simulink model "modelo_matematico"  (R2018b)
settings: Solver=ode4  StartTime=0.0  StopTime=t_f  FixedStep=fst  RelTol=1e-3  EnableMultiTasking=on
values from neighbouring files (symbols this model uses):
  a = plot(dado_t, dado_vd, '-', 'Color',[1.0,0.5,0.0], 'LineWidth', 4)    [Graficos.m]    (also in Trajetoria_Curva_180_graus_RAMPA.m = 0.15)
  b = plot(dado_t, dado_vr, '-', 'Color',[0.0,0.0,0.0], 'LineWidth', 1)    [Graficos.m]    (also in script_principal.m = 0.121)
  c_d = r_d/(2*b)    (= 0.120661157025)    [script_principal.m]
  c_e = r_e/(2*b)    (= 0.121074380165)    [script_principal.m]
  dur_c = dist_c/v    (= 3.5903916041)    [Trajetoria_Curva_180_graus_RAMPA.m]
  k0 = 10    [script_principal.m]
  KaD = 0.4713    [script_principal.m]
  KaD_v = var_KaD*0.4713    (= 0.4713)    [script_principal.m]
  KaE = 0.5046    [script_principal.m]
  KaE_v = var_KaE*0.5046    (= 0.5046)    [script_principal.m]
  L = 0.1    [script_principal.m]
  T = 3    [script_principal.m]
  t_f = t_i+dur_0+dur_1+dur_c+dur_2+dur_3    (= 17.9237249374)    [Trajetoria_Curva_180_graus_RAMPA.m]
  t_i = 0    [Trajetoria_Curva_180_graus_RAMPA.m]
  t_i_1 = t_i+dur_0    (= 2.33333333333)    [Trajetoria_Curva_180_graus_RAMPA.m]
  t_i_2 = t_i+dur_0+dur_1+dur_c    (= 10.7570582708)    [Trajetoria_Curva_180_graus_RAMPA.m]
  t_i_3 = t_i+dur_0+dur_1+dur_c+dur_2    (= 15.5903916041)    [Trajetoria_Curva_180_graus_RAMPA.m]
  t_i_c = t_i+dur_0+dur_1    (= 7.16666666667)    [Trajetoria_Curva_180_graus_RAMPA.m]
  v = 0.35    [Trajetoria_Curva_180_graus_RAMPA.m]
  VaD_max = 14    [script_principal.m]
  VaE_max = 14    [script_principal.m]
  x0 = [x0_1; x0_2; x0_3]    [script_principal.m]
undefined symbols (not defined in the file or in its folder): time_c, w, wx, wy
libraries: simulink x37, dspmtrx3 x2
settings Model: Creator=nenem  LastModifiedBy=nenem
settings OptimizationCC: LifeSpan=inf
settings DebuggingCC: SFUnexpectedBacktrackingDiag=warning  SFNoUnconditionalDefaultTransitionDiag=warning
settings SFSimCC: SimUseLocalCustomCode=off
settings RTWCC: RTWUseLocalCustomCode=off
settings CodeAppCC: StateflowObjectComments=on
settings GRTTargetCC: TargetLangStandard=C89/C90 (ANSI)  GeneratePreprocessorConditionals=Disable all
settings ConfigComp: CovMetricSettings=dw  CovHtmlReporting=on  CovSaveCumulativeToWorkspaceVar=on  CovSaveSingleToWorkspaceVar=on  CovExternalEMLEnable=off

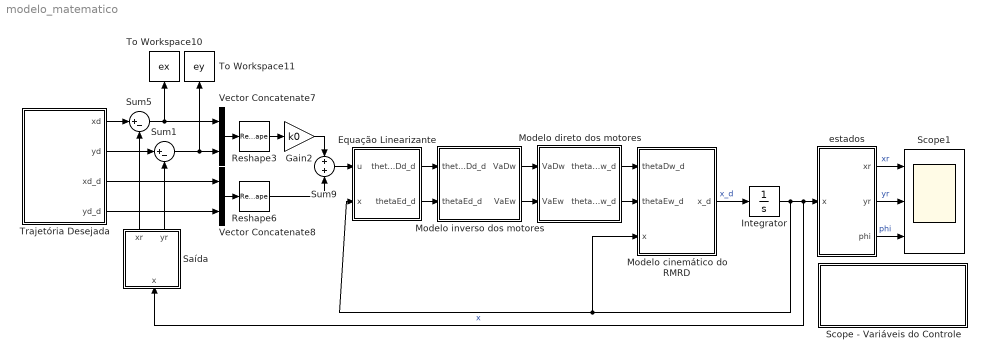
== system modelo_matematico ==
  " Modelo inverso dos motores" : Subsystem
  Equação Linearizante : Subsystem
  Gain2 : Gain  Gain=k0
  Integrator : Integrator  InitialCondition=x0
  Modelo cinemático do RMRD : Subsystem
  Modelo direto dos motores : Subsystem
  Reshape3 : Reshape  OutputDimensionality=Customize  OutputDimensions=[2,1]
  Reshape6 : Reshape  OutputDimensionality=Customize  OutputDimensions=[2,1]
  Saída : Subsystem
  Scope - Variáveis do Controle : Subsystem
  Scope1 : Scope  NumInputPorts=3
  Sum1 : Sum  Inputs=|+-
  Sum5 : Sum  Inputs=|+-
  Sum9 : Sum  Inputs=+|+
  To Workspace10 : ToWorkspace  VariableName=ex  SaveFormat=Structure With Time  SampleTime=-1
      settings: Save2DSignal=2-D array (concatenate along first dimension)
  To Workspace11 : ToWorkspace  VariableName=ey  SaveFormat=Structure With Time  SampleTime=-1
      settings: Save2DSignal=2-D array (concatenate along first dimension)
  Trajetória Desejada : Subsystem
  Vector Concatenate7 : Concatenate
  Vector Concatenate8 : Concatenate
  estados : Subsystem
  wires:
  Modelo cinemático do RMRD/1(x_d) -> Integrator/1  "x_d"
  Integrator/1 -> Modelo cinemático do RMRD/3(x), Equação Linearizante/2(x), estados/1(x), Saída/1(x)  "x"
  Trajetória Desejada/1(xd) -> Sum5/1
  Trajetória Desejada/2(yd) -> Sum1/1
  Trajetória Desejada/4(yd_d) -> Vector Concatenate8/2
  Trajetória Desejada/3(xd_d) -> Vector Concatenate8/1
  Sum5/1 -> To Workspace10/1, Vector Concatenate7/1
  Sum1/1 -> To Workspace11/1, Vector Concatenate7/2
  Gain2/1 -> Sum9/1
  Reshape3/1 -> Gain2/1
  Reshape6/1 -> Sum9/2
  Vector Concatenate7/1 -> Reshape3/1
  Vector Concatenate8/1 -> Reshape6/1
  Sum9/1 -> Equação Linearizante/1(u)
  " Modelo inverso dos motores"/1(VaDw) -> Modelo direto dos motores/1(VaDw)
  " Modelo inverso dos motores"/2(VaEw) -> Modelo direto dos motores/2(VaEw)
  Equação Linearizante/1(thetaDd_d) -> " Modelo inverso dos motores"/1(thetaDd_d)
  Equação Linearizante/2(thetaEd_d) -> " Modelo inverso dos motores"/2(thetaEd_d)
  Modelo direto dos motores/1(thetaDw_d) -> Modelo cinemático do RMRD/1(thetaDw_d)
  Modelo direto dos motores/2(thetaEw_d) -> Modelo cinemático do RMRD/2(thetaEw_d)
  estados/1(xr) -> Scope1/1  "xr"
  estados/3(phi) -> Scope1/3  "phi"
  estados/2(yr) -> Scope1/2  "yr"
  Saída/1(xr) -> Sum5/2
  Saída/2(yr) -> Sum1/2

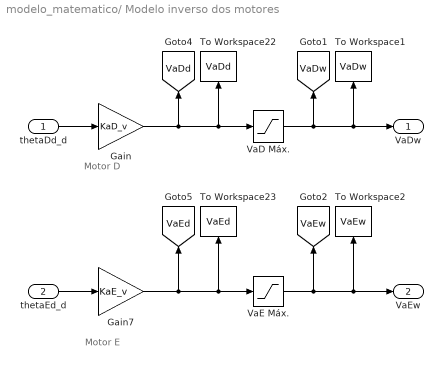
== system modelo_matematico/ Modelo inverso dos motores ==
  note: Motor D
  note: Motor E
  thetaDd_d : Inport
  thetaEd_d : Inport  Port=2
  Gain : Gain  Gain=KaD_v
  Gain7 : Gain  Gain=KaE_v
  To Workspace1 : ToWorkspace  VariableName=VaDw  SaveFormat=Structure With Time  SampleTime=-1
      settings: Save2DSignal=2-D array (concatenate along first dimension)
  To Workspace2 : ToWorkspace  VariableName=VaEw  SaveFormat=Structure With Time  SampleTime=-1
      settings: Save2DSignal=2-D array (concatenate along first dimension)
  To Workspace22 : ToWorkspace  VariableName=VaDd  SaveFormat=Structure With Time  SampleTime=-1
      settings: Save2DSignal=2-D array (concatenate along first dimension)
  To Workspace23 : ToWorkspace  VariableName=VaEd  SaveFormat=Structure With Time  SampleTime=-1
      settings: Save2DSignal=2-D array (concatenate along first dimension)
  VaD Máx. : Saturate  UpperLimit=VaD_max  LowerLimit=-VaD_max
  VaE Máx. : Saturate  UpperLimit=VaE_max  LowerLimit=-VaE_max
  VaDw : Outport
  VaEw : Outport  Port=2
  tag scope: VaDd=global, VaDw=global, VaEd=global, VaEw=global
  wires:
  thetaDd_d/1 -> Gain/1
  thetaEd_d/1 -> Gain7/1
  Gain/1 -> VaD Máx./1, To Workspace22/1, [VaDd]
  Gain7/1 -> [VaEd], To Workspace23/1, VaE Máx./1
  VaE Máx./1 -> VaEw/1, To Workspace2/1, [VaEw]
  VaD Máx./1 -> VaDw/1, To Workspace1/1, [VaDw]

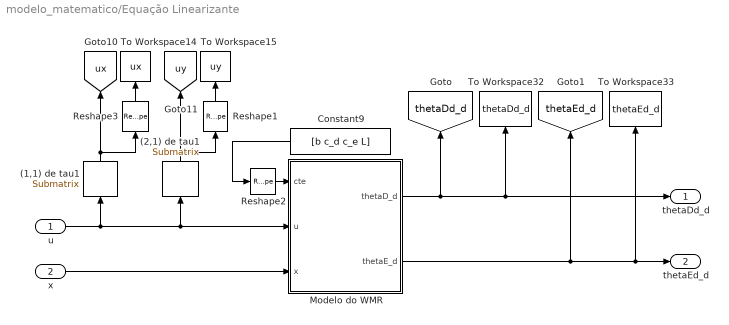
== system modelo_matematico/Equação Linearizante ==
  u : Inport
  x : Inport  Port=2
  (1,1) de tau1 : dspmtrx3/Submatrix  RowSpan=One row  RowStartMode=Index  RowStartIndex=1  RowEndMode=Last  RowEndIndex=1  ColSpan=One column  ColStartMode=Index  ColStartIndex=1  ColEndMode=Last  ColEndIndex=1
  (2,1) de tau1 : dspmtrx3/Submatrix  RowSpan=One row  RowStartMode=Index  RowStartIndex=2  RowEndMode=Last  RowEndIndex=1  ColSpan=One column  ColStartMode=Index  ColStartIndex=1  ColEndMode=Last  ColEndIndex=1
  Constant9 : Constant  Value=[b c_d c_e L]
  Modelo do WMR : MATLAB Function  TreatAsAtomicUnit=on
  Reshape1 : Reshape
  Reshape2 : Reshape  OutputDimensionality=Customize  OutputDimensions=[1,4]
  Reshape3 : Reshape
  To Workspace14 : ToWorkspace  VariableName=ux  SaveFormat=Structure With Time  SampleTime=-1
      settings: Save2DSignal=2-D array (concatenate along first dimension)
  To Workspace15 : ToWorkspace  VariableName=uy  SaveFormat=Structure With Time  SampleTime=-1
      settings: Save2DSignal=2-D array (concatenate along first dimension)
  To Workspace32 : ToWorkspace  VariableName=thetaDd_d  SaveFormat=Structure With Time  SampleTime=-1
      settings: Save2DSignal=2-D array (concatenate along first dimension)
  To Workspace33 : ToWorkspace  VariableName=thetaEd_d  SaveFormat=Structure With Time  SampleTime=-1
      settings: Save2DSignal=2-D array (concatenate along first dimension)
  thetaDd_d : Outport
  thetaEd_d : Outport  Port=2
  tag scope: thetaDd_d=global, thetaEd_d=global, ux=global, uy=global
  wires:
  x/1 -> Modelo do WMR/3(x)
  Reshape2/1 -> Modelo do WMR/1(cte)
  Constant9/1 -> Reshape2/1
  u/1 -> (1,1) de tau1/1, (2,1) de tau1/1, Modelo do WMR/2(u)
  (2,1) de tau1/1 -> [uy], Reshape1/1
  (1,1) de tau1/1 -> [ux], Reshape3/1
  Modelo do WMR/1(thetaD_d) -> [thetaDd_d], To Workspace32/1, thetaDd_d/1
  Modelo do WMR/2(thetaE_d) -> thetaEd_d/1, To Workspace33/1, [thetaEd_d]
  Reshape1/1 -> To Workspace15/1
  Reshape3/1 -> To Workspace14/1

== system modelo_matematico/Modelo cinemático do RMRD ==
  thetaDw_d : Inport
  thetaEw_d : Inport  Port=2
  x : Inport  Port=3
  Constant9 : Constant  Value=[b c_d c_e L]
  Modelo do RMRD : MATLAB Function  TreatAsAtomicUnit=on
  Reshape2 : Reshape  OutputDimensionality=Customize  OutputDimensions=[1,4]
  x_d : Outport
  wires:
  x/1 -> Modelo do RMRD/4(x)
  thetaEw_d/1 -> Modelo do RMRD/3(thetaE_d)
  thetaDw_d/1 -> Modelo do RMRD/2(thetaD_d)
  Reshape2/1 -> Modelo do RMRD/1(cte)
  Constant9/1 -> Reshape2/1
  Modelo do RMRD/1(x_d) -> x_d/1  "x_d"

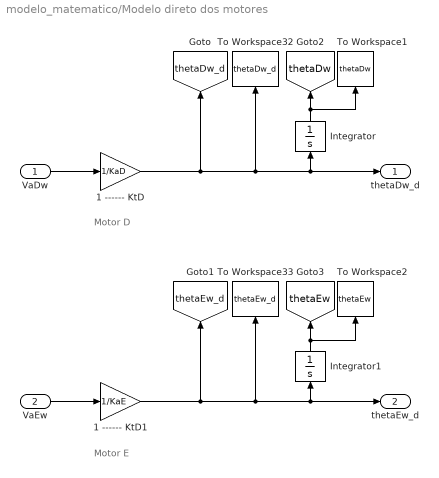
== system modelo_matematico/Modelo direto dos motores ==
  note: Motor D
  note: Motor E
  VaDw : Inport
  VaEw : Inport  Port=2
  1 ------ KtD : Gain  Gain=1/KaD
  1 ------ KtD1 : Gain  Gain=1/KaE
  Integrator : Integrator
  Integrator1 : Integrator
  To Workspace1 : ToWorkspace  VariableName=thetaDw  SaveFormat=Structure With Time  SampleTime=-1
      settings: Save2DSignal=2-D array (concatenate along first dimension)
  To Workspace2 : ToWorkspace  VariableName=thetaEw  SaveFormat=Structure With Time  SampleTime=-1
      settings: Save2DSignal=2-D array (concatenate along first dimension)
  To Workspace32 : ToWorkspace  VariableName=thetaDw_d  SaveFormat=Structure With Time  SampleTime=-1
      settings: Save2DSignal=2-D array (concatenate along first dimension)
  To Workspace33 : ToWorkspace  VariableName=thetaEw_d  SaveFormat=Structure With Time  SampleTime=-1
      settings: Save2DSignal=2-D array (concatenate along first dimension)
  thetaDw_d : Outport
  thetaEw_d : Outport  Port=2
  tag scope: thetaDw=global, thetaDw_d=global, thetaEw=global, thetaEw_d=global
  wires:
  1 ------ KtD/1 -> [thetaDw_d], thetaDw_d/1, Integrator/1, To Workspace32/1
  1 ------ KtD1/1 -> [thetaEw_d], thetaEw_d/1, Integrator1/1, To Workspace33/1
  Integrator/1 -> To Workspace1/1, [thetaDw]
  Integrator1/1 -> To Workspace2/1, [thetaEw]
  VaDw/1 -> 1 ------ KtD/1
  VaEw/1 -> 1 ------ KtD1/1

== system modelo_matematico/Saída ==
  x : Inport
  Derivative : Derivative
  Derivative1 : Derivative
  Hypot2 : Math  Operator=hypot  SaturateOnIntegerOverflow=on
  Reshape1 : Reshape  OutputDimensionality=Customize  OutputDimensions=[3,1]
  Saídas : MATLAB Function  TreatAsAtomicUnit=on
  To Workspace1 : ToWorkspace  VariableName=xr_d  SaveFormat=Structure With Time  SampleTime=-1
      settings: Save2DSignal=2-D array (concatenate along first dimension)
  To Workspace2 : ToWorkspace  VariableName=yr_d  SaveFormat=Structure With Time  SampleTime=-1
      settings: Save2DSignal=2-D array (concatenate along first dimension)
  To Workspace7 : ToWorkspace  VariableName=vr  SaveFormat=Structure With Time  SampleTime=-1
      settings: Save2DSignal=2-D array (concatenate along first dimension)
  xr : Outport
  yr : Outport  Port=2
  wires:
  x/1 -> Reshape1/1
  Saídas/1(xr) -> Derivative/1, xr/1
  Saídas/2(yr) -> yr/1, Derivative1/1
  Hypot2/1 -> To Workspace7/1
  Derivative/1 -> To Workspace1/1, Hypot2/2
  Derivative1/1 -> Hypot2/1, To Workspace2/1
  Reshape1/1 -> Saídas/1(x)

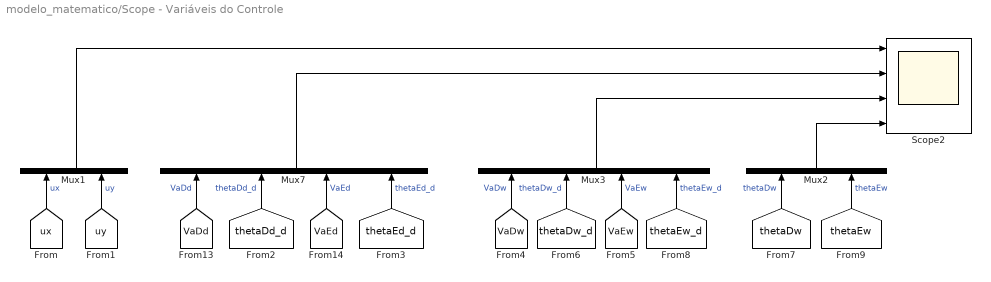
== system modelo_matematico/Scope - Variáveis do Controle ==
  Mux1 : Mux  Inputs=2
  Mux2 : Mux  Inputs=2
  Mux3 : Mux
  Mux7 : Mux
  Scope2 : Scope  NumInputPorts=4
  wires:
  [thetaEw_d] -> Mux3/4  "thetaEw_d"
  Mux3/1 -> Scope2/3
  [thetaDw_d] -> Mux3/2  "thetaDw_d"
  [VaEw] -> Mux3/3  "VaEw"
  [VaDw] -> Mux3/1  "VaDw"
  [thetaEd_d] -> Mux7/4  "thetaEd_d"
  [thetaDd_d] -> Mux7/2  "thetaDd_d"
  Mux7/1 -> Scope2/2
  Mux1/1 -> Scope2/1
  [ux] -> Mux1/1  "ux"
  [uy] -> Mux1/2  "uy"
  [VaDd] -> Mux7/1  "VaDd"
  [VaEd] -> Mux7/3  "VaEd"
  [thetaDw] -> Mux2/1  "thetaDw"
  [thetaEw] -> Mux2/2  "thetaEw"
  Mux2/1 -> Scope2/4

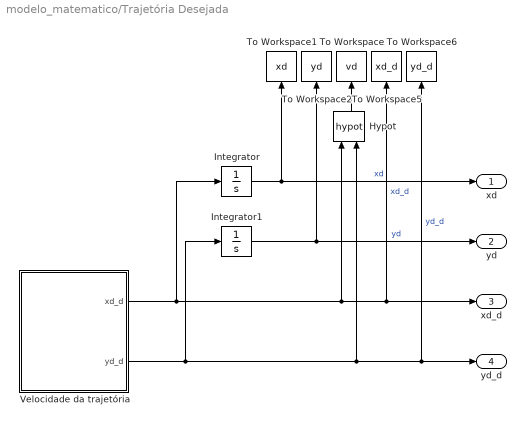
== system modelo_matematico/Trajetória Desejada ==
  Hypot : Math  Operator=hypot  OutputSignalType=real  SaturateOnIntegerOverflow=on
  Integrator : Integrator
  Integrator1 : Integrator
  To Workspace : ToWorkspace  VariableName=vd  SaveFormat=Structure With Time  SampleTime=-1
      settings: Save2DSignal=2-D array (concatenate along first dimension)
  To Workspace1 : ToWorkspace  VariableName=xd  SaveFormat=Structure With Time  SampleTime=-1
      settings: Save2DSignal=2-D array (concatenate along first dimension)
  To Workspace2 : ToWorkspace  VariableName=yd  SaveFormat=Structure With Time  SampleTime=-1
      settings: Save2DSignal=2-D array (concatenate along first dimension)
  To Workspace5 : ToWorkspace  VariableName=xd_d  SaveFormat=Structure With Time  SampleTime=-1
      settings: Save2DSignal=2-D array (concatenate along first dimension)
  To Workspace6 : ToWorkspace  VariableName=yd_d  SaveFormat=Structure With Time  SampleTime=-1
      settings: Save2DSignal=2-D array (concatenate along first dimension)
  Velocidade da trajetória : Subsystem
  xd : Outport
  yd : Outport  Port=2
  xd_d : Outport  Port=3
  yd_d : Outport  Port=4
  wires:
  Integrator/1 -> xd/1, To Workspace1/1  "xd"
  Integrator1/1 -> yd/1, To Workspace2/1  "yd"
  Hypot/1 -> To Workspace/1
  Velocidade da trajetória/1(xd_d) -> Integrator/1, xd_d/1, To Workspace5/1, Hypot/1  "xd_d"
  Velocidade da trajetória/2(yd_d) -> Integrator1/1, yd_d/1, To Workspace6/1, Hypot/2  "yd_d"

== system modelo_matematico/estados ==
  x : Inport
  Estados : MATLAB Function  TreatAsAtomicUnit=on
  To Workspace2 : ToWorkspace  VariableName=phi  SaveFormat=Structure With Time  SampleTime=-1
      settings: Save2DSignal=2-D array (concatenate along first dimension)
  To Workspace3 : ToWorkspace  VariableName=xr  SaveFormat=Structure With Time  SampleTime=-1
      settings: Save2DSignal=2-D array (concatenate along first dimension)
  To Workspace4 : ToWorkspace  VariableName=yr  SaveFormat=Structure With Time  SampleTime=-1
      settings: Save2DSignal=2-D array (concatenate along first dimension)
  xr : Outport
  yr : Outport  Port=2
  phi : Outport  Port=3
  wires:
  x/1 -> Estados/1(x)
  Estados/1(xr) -> xr/1, To Workspace3/1
  Estados/2(yr) -> yr/1, To Workspace4/1
  Estados/3(phi) -> phi/1, To Workspace2/1

== system modelo_matematico/Trajetória Desejada/Velocidade da trajetória ==
  0 : Subsystem  Commented=on
  0 c/ RAMPA : Subsystem  Commented=on
  180 c/ RAMPA : Subsystem
  8 : Subsystem  Commented=on
  "90 " : Subsystem  Commented=on
  90 c/ RAMPA : Subsystem  Commented=on
  Constant : Constant  Value=T
  Multiport Switch : MultiPortSwitch  Inputs=4
  Multiport Switch1 : MultiPortSwitch  Inputs=4
  Reta c/ RAMPA : Subsystem  Commented=on
  xd_d : Outport
  yd_d : Outport  Port=2
  wires:
  0 c/ RAMPA/2(yd_d) -> Multiport Switch1/2  "yd_d"
  90 c/ RAMPA/2(yd_d) -> Multiport Switch1/3  "yd_d"
  90 c/ RAMPA/1(xd_d) -> Multiport Switch/3  "xd_d"
  0 c/ RAMPA/1(xd_d) -> Multiport Switch/2  "xd_d"
  Constant/1 -> Multiport Switch/1, Multiport Switch1/1
  Multiport Switch/1 -> xd_d/1  "xd_d"
  Multiport Switch1/1 -> yd_d/1  "yd_d"
  8/2(yd_d) -> Multiport Switch1/5  "yd_d"
  180 c/ RAMPA/2(yd_d) -> Multiport Switch1/4  "yd_d"
  180 c/ RAMPA/1(xd_d) -> Multiport Switch/4  "xd_d"
  8/1(xd_d) -> Multiport Switch/5

== system modelo_matematico/Trajetória Desejada/Velocidade da trajetória/0 ==
  Gain : Gain  Gain=w
  Gain1 : Gain  Gain=v
  Gain2 : Gain  Gain=w
  Gain3 : Gain  Gain=v
  Gain4 : Gain  Gain=-1
  Ramp18 : simulink/Sources/Ramp  slope=1  start=t_i  InitialOutput=0
  Ramp19 : simulink/Sources/Ramp  slope=-1  start=t_i  InitialOutput=0
  Trigonometric Function : Trigonometry
  Trigonometric Function1 : Trigonometry  Operator=cos
  xd_d : Outport
  yd_d : Outport  Port=2
  wires:
  Gain4/1 -> Gain1/1
  Ramp18/1 -> Gain/1
  Gain/1 -> Trigonometric Function/1
  Trigonometric Function1/1 -> Gain3/1
  Gain2/1 -> Trigonometric Function1/1
  Ramp19/1 -> Gain2/1
  Gain1/1 -> xd_d/1
  Gain3/1 -> yd_d/1
  Trigonometric Function/1 -> Gain4/1

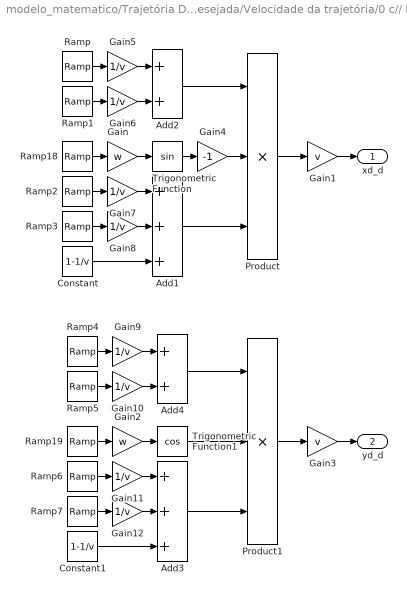
== system modelo_matematico/Trajetória Desejada/Velocidade da trajetória/0 c// RAMPA ==
  Add1 : Sum  Inputs=3
  Add2 : Sum  Inputs=2
  Add3 : Sum  Inputs=3
  Add4 : Sum  Inputs=2
  Constant : Constant  Value=1-1/v
  Constant1 : Constant  Value=1-1/v
  Gain : Gain  Gain=w
  Gain1 : Gain  Gain=v
  Gain{5..12} (8 alike) : Gain  Gain=1/v
  Gain2 : Gain  Gain=w
  Gain3 : Gain  Gain=v
  Gain4 : Gain  Gain=-1
  Product : Product  Inputs=3
  Product1 : Product  Inputs=3
  Ramp : simulink/Sources/Ramp  slope=a  start=t_i  InitialOutput=0
  Ramp1 : simulink/Sources/Ramp  slope=-a  start=t_1  InitialOutput=0
  Ramp18 : simulink/Sources/Ramp  slope=1  start=t_i  InitialOutput=0
  Ramp19 : simulink/Sources/Ramp  slope=1  start=t_i  InitialOutput=0
  Ramp2 : simulink/Sources/Ramp  slope=-a  start=t_2  InitialOutput=1
  Ramp3 : simulink/Sources/Ramp  slope=a  start=t_f  InitialOutput=0
  Ramp4 : simulink/Sources/Ramp  slope=a  start=t_i  InitialOutput=0
  Ramp5 : simulink/Sources/Ramp  slope=-a  start=t_1  InitialOutput=0
  Ramp6 : simulink/Sources/Ramp  slope=-a  start=t_2  InitialOutput=1
  Ramp7 : simulink/Sources/Ramp  slope=a  start=t_f  InitialOutput=0
  Trigonometric Function : Trigonometry
  Trigonometric Function1 : Trigonometry  Operator=cos
  xd_d : Outport
  yd_d : Outport  Port=2
  wires:
  Product/1 -> Gain1/1
  Ramp18/1 -> Gain/1
  Gain/1 -> Trigonometric Function/1
  Gain2/1 -> Trigonometric Function1/1
  Ramp19/1 -> Gain2/1
  Gain1/1 -> xd_d/1
  Gain3/1 -> yd_d/1
  Trigonometric Function/1 -> Gain4/1
  Ramp/1 -> Gain5/1
  Ramp1/1 -> Gain6/1
  Gain5/1 -> Add2/1
  Gain6/1 -> Add2/2
  Add2/1 -> Product/1
  Gain4/1 -> Product/2
  Product1/1 -> Gain3/1
  Trigonometric Function1/1 -> Product1/2
  Ramp2/1 -> Gain7/1
  Gain7/1 -> Add1/1
  Ramp3/1 -> Gain8/1
  Gain8/1 -> Add1/2
  Add1/1 -> Product/3
  Constant/1 -> Add1/3
  Ramp6/1 -> Gain11/1
  Add3/1 -> Product1/3
  Constant1/1 -> Add3/3
  Gain12/1 -> Add3/2
  Gain9/1 -> Add4/1
  Add4/1 -> Product1/1
  Gain11/1 -> Add3/1
  Ramp4/1 -> Gain9/1
  Ramp7/1 -> Gain12/1
  Gain10/1 -> Add4/2
  Ramp5/1 -> Gain10/1

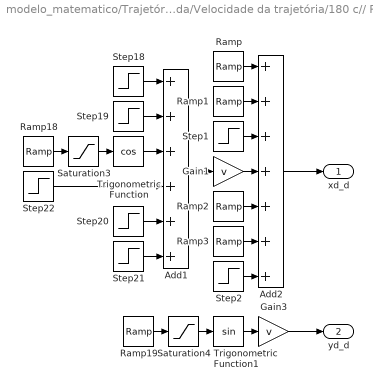
== system modelo_matematico/Trajetória Desejada/Velocidade da trajetória/180 c// RAMPA ==
  Add1 : Sum  Inputs=++++++
  Add2 : Sum  Inputs=+++++++
  Gain1 : Gain  Gain=v
  Gain3 : Gain  Gain=v
  Ramp : simulink/Sources/Ramp  slope=a  start=t_i  InitialOutput=0
  Ramp1 : simulink/Sources/Ramp  slope=-a  start=t_i_1  InitialOutput=0
  Ramp18 : simulink/Sources/Ramp  slope=pi/dur_c  start=t_i_c  InitialOutput=0
  Ramp19 : simulink/Sources/Ramp  slope=pi/dur_c  start=t_i_c  InitialOutput=0
  Ramp2 : simulink/Sources/Ramp  slope=a  start=t_i_3  InitialOutput=0
  Ramp3 : simulink/Sources/Ramp  slope=-a  start=t_f  InitialOutput=0
  Saturation3 : Saturate  UpperLimit=pi  LowerLimit=0
  Saturation4 : Saturate  UpperLimit=pi  LowerLimit=0
  Step1 : Step  Time=t_i_1  After=-v  SampleTime=0
  Step18 : Step  Time=t_i_1  SampleTime=0
  Step19 : Step  Time=t_i_c  After=-1  SampleTime=0
  Step2 : Step  Time=t_i_3  After=-v  SampleTime=0
  Step20 : Step  Time=t_i_3  SampleTime=0
  Step21 : Step  Time=t_f  After=-1  SampleTime=0
  Step22 : Step  Time=t_i_c  Before=-1  After=0  SampleTime=0
  Trigonometric Function : Trigonometry  Operator=cos
  Trigonometric Function1 : Trigonometry
  xd_d : Outport
  yd_d : Outport  Port=2
  wires:
  Add1/1 -> Gain1/1
  Ramp18/1 -> Saturation3/1
  Saturation3/1 -> Trigonometric Function/1
  Saturation4/1 -> Trigonometric Function1/1
  Ramp19/1 -> Saturation4/1
  Step18/1 -> Add1/1
  Step19/1 -> Add1/2
  Trigonometric Function/1 -> Add1/3
  Step22/1 -> Add1/4
  Add2/1 -> xd_d/1
  Ramp/1 -> Add2/1
  Ramp1/1 -> Add2/2
  Step1/1 -> Add2/3
  Gain1/1 -> Add2/4
  Gain3/1 -> yd_d/1
  Ramp2/1 -> Add2/5
  Ramp3/1 -> Add2/6
  Step20/1 -> Add1/5
  Step21/1 -> Add1/6
  Step2/1 -> Add2/7
  Trigonometric Function1/1 -> Gain3/1

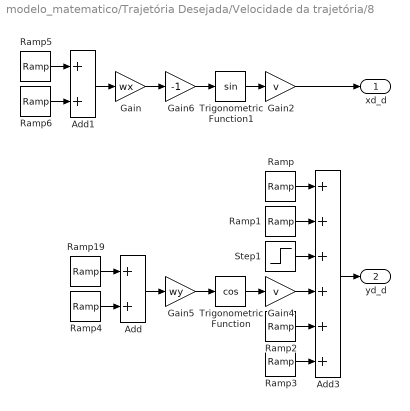
== system modelo_matematico/Trajetória Desejada/Velocidade da trajetória/8 ==
  Add : Sum
  Add1 : Sum
  Add3 : Sum  Inputs=++++++
  Gain : Gain  Gain=wx
  Gain2 : Gain  Gain=v
  Gain4 : Gain  Gain=v
  Gain5 : Gain  Gain=wy
  Gain6 : Gain  Gain=-1
  Ramp : simulink/Sources/Ramp  slope=a  start=t_i  InitialOutput=0
  Ramp1 : simulink/Sources/Ramp  slope=-a  start=t_i_1  InitialOutput=0
  Ramp19 : simulink/Sources/Ramp  slope=1  start=t_i_1  InitialOutput=0
  Ramp2 : simulink/Sources/Ramp  slope=-a  start=t_i_2  InitialOutput=0
  Ramp3 : simulink/Sources/Ramp  slope=a  start=t_f  InitialOutput=0
  Ramp4 : simulink/Sources/Ramp  slope=-1  start=t_i_2  InitialOutput=0
  Ramp5 : simulink/Sources/Ramp  slope=1  start=t_i_1  InitialOutput=0
  Ramp6 : simulink/Sources/Ramp  slope=-1  start=t_i_2  InitialOutput=0
  Step1 : Step  Time=t_i  After=-v  SampleTime=0
  Trigonometric Function : Trigonometry  Operator=cos
  Trigonometric Function1 : Trigonometry
  xd_d : Outport
  yd_d : Outport  Port=2
  wires:
  Add1/1 -> Gain/1
  Trigonometric Function/1 -> Gain4/1
  Trigonometric Function1/1 -> Gain2/1
  Add3/1 -> yd_d/1
  Gain/1 -> Gain6/1
  Gain5/1 -> Trigonometric Function/1
  Gain6/1 -> Trigonometric Function1/1
  Gain4/1 -> Add3/4
  Ramp2/1 -> Add3/5
  Ramp3/1 -> Add3/6
  Ramp1/1 -> Add3/2
  Ramp/1 -> Add3/1
  Step1/1 -> Add3/3
  Ramp19/1 -> Add/1
  Add/1 -> Gain5/1
  Ramp4/1 -> Add/2
  Ramp6/1 -> Add1/2
  Ramp5/1 -> Add1/1
  Gain2/1 -> xd_d/1

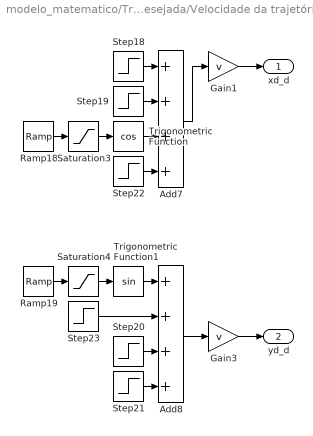
== system modelo_matematico/Trajetória Desejada/Velocidade da trajetória/90  ==
  Add7 : Sum  Inputs=++++
  Add8 : Sum  Inputs=++++
  Gain1 : Gain  Gain=v
  Gain3 : Gain  Gain=v
  Ramp18 : simulink/Sources/Ramp  slope=(pi/2)/time_c  start=t_i_c  InitialOutput=0
  Ramp19 : simulink/Sources/Ramp  slope=(pi/2)/time_c  start=t_i_c  InitialOutput=0
  Saturation3 : Saturate  UpperLimit=pi/2  LowerLimit=0
  Saturation4 : Saturate  UpperLimit=pi/2  LowerLimit=0
  Step18 : Step  Time=t_i  SampleTime=0
  Step19 : Step  Time=t_i_c  After=-1  SampleTime=0
  Step20 : Step  Time=t_i_2  SampleTime=0
  Step21 : Step  Time=t_f  After=-1  SampleTime=0
  Step22 : Step  Time=t_i_c  Before=-1  After=0  SampleTime=0
  Step23 : Step  Time=t_i_2  After=-1  SampleTime=0
  Trigonometric Function : Trigonometry  Operator=cos
  Trigonometric Function1 : Trigonometry
  xd_d : Outport
  yd_d : Outport  Port=2
  wires:
  Add7/1 -> Gain1/1
  Ramp18/1 -> Saturation3/1
  Step21/1 -> Add8/4
  Saturation3/1 -> Trigonometric Function/1
  Add8/1 -> Gain3/1
  Step20/1 -> Add8/3
  Trigonometric Function1/1 -> Add8/1
  Saturation4/1 -> Trigonometric Function1/1
  Ramp19/1 -> Saturation4/1
  Step23/1 -> Add8/2
  Gain1/1 -> xd_d/1
  Gain3/1 -> yd_d/1
  Step22/1 -> Add7/4
  Trigonometric Function/1 -> Add7/3
  Step19/1 -> Add7/2
  Step18/1 -> Add7/1

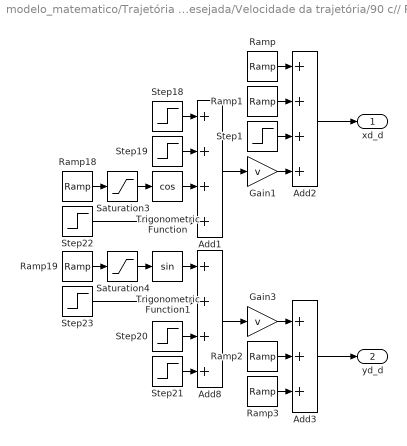
== system modelo_matematico/Trajetória Desejada/Velocidade da trajetória/90 c// RAMPA ==
  Add1 : Sum  Inputs=++++
  Add2 : Sum  Inputs=++++
  Add3 : Sum  Inputs=+++
  Add8 : Sum  Inputs=++++
  Gain1 : Gain  Gain=v
  Gain3 : Gain  Gain=v
  Ramp : simulink/Sources/Ramp  slope=a  start=t_i  InitialOutput=0
  Ramp1 : simulink/Sources/Ramp  slope=-a  start=t_i_1  InitialOutput=0
  Ramp18 : simulink/Sources/Ramp  slope=(pi/2)/dur_c  start=t_i_c  InitialOutput=0
  Ramp19 : simulink/Sources/Ramp  slope=(pi/2)/dur_c  start=t_i_c  InitialOutput=0
  Ramp2 : simulink/Sources/Ramp  slope=-a  start=t_i_3  InitialOutput=0
  Ramp3 : simulink/Sources/Ramp  slope=a  start=t_f  InitialOutput=0
  Saturation3 : Saturate  UpperLimit=pi/2  LowerLimit=0
  Saturation4 : Saturate  UpperLimit=pi/2  LowerLimit=0
  Step1 : Step  Time=t_i_1  After=-v  SampleTime=0
  Step18 : Step  Time=t_i_1  SampleTime=0
  Step19 : Step  Time=t_i_c  After=-1  SampleTime=0
  Step20 : Step  Time=t_i_2  SampleTime=0
  Step21 : Step  Time=t_f  After=-1  SampleTime=0
  Step22 : Step  Time=t_i_c  Before=-1  After=0  SampleTime=0
  Step23 : Step  Time=t_i_2  After=-1  SampleTime=0
  Trigonometric Function : Trigonometry  Operator=cos
  Trigonometric Function1 : Trigonometry
  xd_d : Outport
  yd_d : Outport  Port=2
  wires:
  Add1/1 -> Gain1/1
  Ramp18/1 -> Saturation3/1
  Step21/1 -> Add8/4
  Saturation3/1 -> Trigonometric Function/1
  Add8/1 -> Gain3/1
  Step20/1 -> Add8/3
  Trigonometric Function1/1 -> Add8/1
  Saturation4/1 -> Trigonometric Function1/1
  Ramp19/1 -> Saturation4/1
  Step23/1 -> Add8/2
  Step18/1 -> Add1/1
  Step19/1 -> Add1/2
  Trigonometric Function/1 -> Add1/3
  Step22/1 -> Add1/4
  Add2/1 -> xd_d/1
  Ramp/1 -> Add2/1
  Ramp1/1 -> Add2/2
  Step1/1 -> Add2/3
  Gain1/1 -> Add2/4
  Gain3/1 -> Add3/1
  Add3/1 -> yd_d/1
  Ramp2/1 -> Add3/2
  Ramp3/1 -> Add3/3

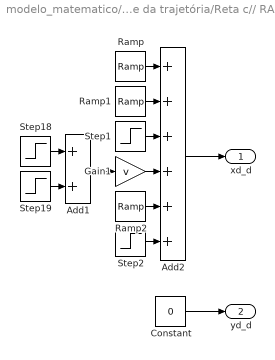
== system modelo_matematico/Trajetória Desejada/Velocidade da trajetória/Reta c// RAMPA ==
  Add1 : Sum
  Add2 : Sum  Inputs=++++++
  Constant : Constant  Value=0
  Gain1 : Gain  Gain=v
  Ramp : simulink/Sources/Ramp  slope=a  start=t_i  InitialOutput=0
  Ramp1 : simulink/Sources/Ramp  slope=-a  start=t_i_1  InitialOutput=0
  Ramp2 : simulink/Sources/Ramp  slope=-a  start=t_i_2  InitialOutput=0
  Step1 : Step  Time=t_i_1  After=-v  SampleTime=0
  Step18 : Step  Time=t_i_1  SampleTime=0
  Step19 : Step  Time=t_i_2  After=-1  SampleTime=0
  Step2 : Step  Time=t_i_2  After=v  SampleTime=0
  xd_d : Outport
  yd_d : Outport  Port=2
  wires:
  Add1/1 -> Gain1/1
  Step18/1 -> Add1/1
  Step19/1 -> Add1/2
  Add2/1 -> xd_d/1
  Ramp/1 -> Add2/1
  Ramp1/1 -> Add2/2
  Step1/1 -> Add2/3
  Gain1/1 -> Add2/4
  Ramp2/1 -> Add2/5
  Step2/1 -> Add2/6
  Constant/1 -> yd_d/1

== matlab function modelo_matematico/Equação Linearizante/Modelo do WMR ==
  data: cte input; u input; x input; thetaD_d output; thetaE_d output
function [thetaD_d, thetaE_d] = fcn(cte, u, x)
%#codegen
% Parametros de simulação--------------------------------------------------
b   = cte(1,1);
c_d = cte(1,2);
c_e = cte(1,3);
L   = cte(1,4);

phi = x(3,1);

% Cálculo de D e u---------------------------------------------------------
D = [c_d*b*cos(phi)-c_d*L*sin(phi) c_e*b*cos(phi)+c_e*L*sin(phi);
     c_d*b*sin(phi)+c_d*L*cos(phi) c_e*b*sin(phi)-c_e*L*cos(phi)];

eta = D^-1*(u);
 
% Cálculo de x_d-----------------------------------------------------------
thetaD_d = eta(1,1);
thetaE_d = eta(2,1);

== matlab function modelo_matematico/Modelo cinemático do RMRD/Modelo do RMRD ==
  data: cte input; thetaD_d input; thetaE_d input; x input; x_d output
function x_d = fcn(cte, thetaD_d, thetaE_d, x)
%#codegen
% Parametros de simulação--------------------------------------------------
b   = cte(1,1);
c_d = cte(1,2);
c_e = cte(1,3);
L   = cte(1,4);

phi = x(3,1);

% Cálculo de D e u---------------------------------------------------------
J = [c_d*b*cos(phi)-L*c_d*sin(phi), c_e*b*cos(phi)+L*c_e*sin(phi);
     c_d*b*sin(phi)+L*c_d*cos(phi), c_e*b*sin(phi)-L*c_e*cos(phi);
                               c_d,                          -c_e];
eta = [thetaD_d;
       thetaE_d];
 
% Cálculo de x_d-----------------------------------------------------------
x_d = J*eta;

== matlab function modelo_matematico/estados/Estados ==
  data: xr output; yr output; x input; phi output
function [xr, yr, phi] = fcn(x)

%#codegen
%--------------------------------------------------------------------------
xr  = x(1,1);
yr  = x(2,1);
phi = x(3,1);

== matlab function modelo_matematico/Saída/Saídas ==
  data: xr output; yr output; x input
function [xr, yr] = fcn(x)

%#codegen
xr     = x(1,1);
yr     = x(2,1);
